simulink model "Z_Feedback"  (R2022b)
settings: Solver=FixedStepAuto  StartTime=0.0  StopTime=10.0  FixedStep=step_size  RelTol=1e-3
undefined symbols (not defined in the file): unicycle
libraries: simulink_extras x1
settings Model: Creator=Musta  LastModifiedBy=mustacchim

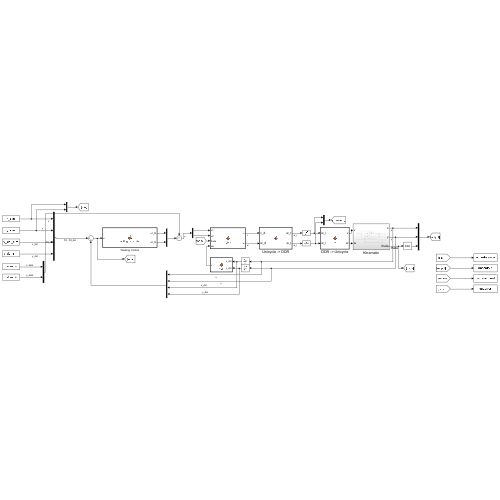
[thumbnail: Simulink's stored preview of the top-level diagram]
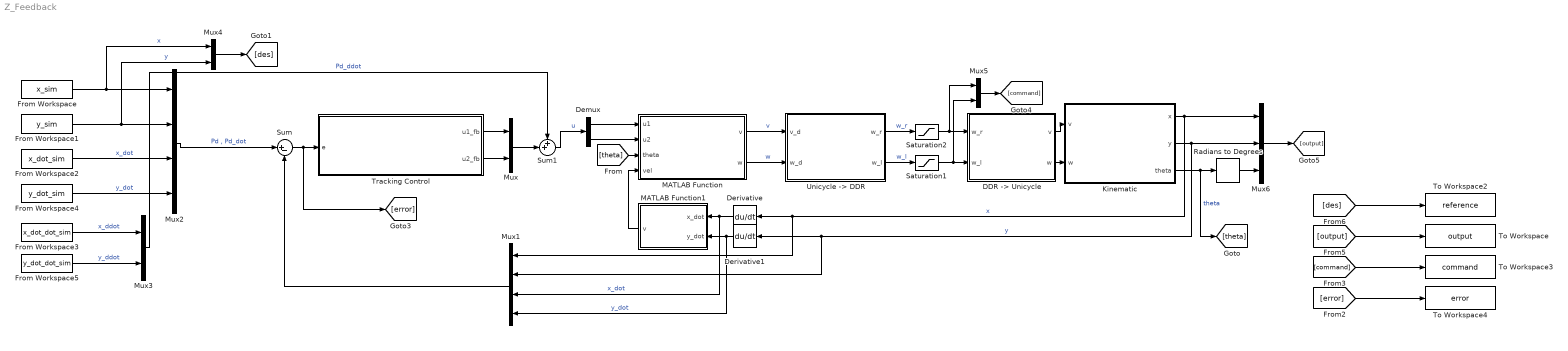
== system Z_Feedback ==
  " DDR -> Unicycle " : MATLAB Function  TreatAsAtomicUnit=on
  Demux : Demux  Outputs=2
  Derivative : Derivative
  Derivative1 : Derivative
  From Workspace : FromWorkspace  VariableName=x_sim
  From Workspace1 : FromWorkspace  VariableName=y_sim
  From Workspace2 : FromWorkspace  VariableName=x_dot_sim
  From Workspace3 : FromWorkspace  VariableName=x_dot_dot_sim
  From Workspace4 : FromWorkspace  VariableName=y_dot_sim
  From Workspace5 : FromWorkspace  VariableName=y_dot_dot_sim
  Kinematic : Subsystem
  MATLAB Function : MATLAB Function  TreatAsAtomicUnit=on
  MATLAB Function1 : MATLAB Function  TreatAsAtomicUnit=on
  Mux{,3..5} (4 alike) : Mux  Inputs=2
  Mux1 : Mux
  Mux2 : Mux
  Mux6 : Mux  Inputs=3
  Radians to Degrees : simulink_extras/Transformations/Radians to Degrees
  Saturation1 : Saturate  UpperLimit=unicycle.omegaWheelMax  LowerLimit=unicycle.omegaWheelMin
  Saturation2 : Saturate  UpperLimit=unicycle.omegaWheelMax  LowerLimit=unicycle.omegaWheelMin
  Sum : Sum  Inputs=|+-
  Sum1 : Sum  Inputs=++|
  To Workspace : ToWorkspace  VariableName=output  SaveFormat=Structure With Time  SampleTime=-1
  To Workspace2 : ToWorkspace  VariableName=reference  SaveFormat=Structure With Time  SampleTime=-1
  To Workspace3 : ToWorkspace  VariableName=command  SaveFormat=Structure With Time  SampleTime=-1
  To Workspace4 : ToWorkspace  VariableName=error  SaveFormat=Structure With Time  SampleTime=-1
  Tracking Control : MATLAB Function  TreatAsAtomicUnit=on
  "Unicycle -> DDR" : MATLAB Function  TreatAsAtomicUnit=on
  wires:
  Mux4/1 -> [des]
  Mux1/1 -> Sum/2
  Mux2/1 -> Sum/1  "Pd , Pd_dot"
  Demux/1 -> MATLAB Function/1(u1)
  Mux/1 -> Sum1/2
  Derivative1/1 -> Mux1/4, MATLAB Function1/2(y_dot)  "y_dot"
  From Workspace5/1 -> Mux3/2  "y_ddot"
  Derivative/1 -> Mux1/3, MATLAB Function1/1(x_dot)  "x_dot"
  Demux/2 -> MATLAB Function/2(u2)
  Tracking Control/2(u2_fb) -> Mux/2
  From Workspace1/1 -> Mux2/2, Mux4/2  "y"
  MATLAB Function1/1(v) -> MATLAB Function/4(vel)
  From Workspace3/1 -> Mux3/1  "x_ddot"
  Tracking Control/1(u1_fb) -> Mux/1
  MATLAB Function/1(v) -> "Unicycle -> DDR"/1(v_d)  "v"
  Sum1/1 -> Demux/1  "u"
  MATLAB Function/2(w) -> "Unicycle -> DDR"/2(w_d)  "w"
  From Workspace/1 -> Mux4/1, Mux2/1  "x"
  From Workspace2/1 -> Mux2/3  "x_dot"
  From Workspace4/1 -> Mux2/4  "y_dot"
  Mux3/1 -> Sum1/1  "Pd_ddot"
  Kinematic/3(theta) -> [theta], Radians to Degrees/1  "theta"
  Kinematic/1(x) -> Mux1/1, Derivative/1, Mux6/1  "x"
  " DDR -> Unicycle "/1(v) -> Kinematic/1(v)
  Radians to Degrees/1 -> Mux6/3
  Saturation2/1 -> " DDR -> Unicycle "/1(w_r), Mux5/1
  "Unicycle -> DDR"/1(w_r) -> Saturation2/1  "w_r"
  "Unicycle -> DDR"/2(w_l) -> Saturation1/1  "w_l"
  " DDR -> Unicycle "/2(w) -> Kinematic/2(w)
  Mux6/1 -> [output]
  Saturation1/1 -> Mux5/2, " DDR -> Unicycle "/2(w_l)
  Kinematic/2(y) -> Mux1/2, Derivative1/1, Mux6/2  "y"
  Mux5/1 -> [command]
  Sum/1 -> [error], Tracking Control/1(e)
  [theta] -> MATLAB Function/3(theta)
  [command] -> To Workspace3/1
  [output] -> To Workspace/1
  [des] -> To Workspace2/1
  [error] -> To Workspace4/1

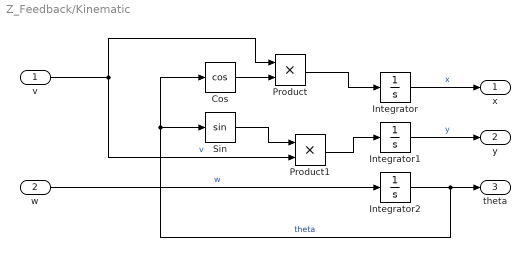
== system Z_Feedback/Kinematic ==
  v : Inport
  w : Inport  Port=2
  Cos : Trigonometry  Operator=cos
  Integrator : Integrator  InitialCondition=unicycle.ic.x
  Integrator1 : Integrator  InitialCondition=unicycle.ic.y
  Integrator2 : Integrator  InitialCondition=unicycle.ic.theta
  Product : Product
  Product1 : Product
  Sin : Trigonometry
  x : Outport
  y : Outport  Port=2
  theta : Outport  Port=3
  wires:
  w/1 -> Integrator2/1  "w"
  Product/1 -> Integrator/1
  v/1 -> Product/1, Product1/2  "v"
  Cos/1 -> Product/2
  Integrator1/1 -> y/1  "y"
  Integrator/1 -> x/1  "x"
  Integrator2/1 -> Cos/1, Sin/1, theta/1  "theta"
  Product1/1 -> Integrator1/1
  Sin/1 -> Product1/1

== matlab function Z_Feedback/MATLAB Function ==
  data: u1 input; u2 input; theta input; v output; w output; vel input
function [v,w] = T_inv(u1,u2,theta,vel)


if abs(vel) < 1e-3
    if abs(vel) >= 0
        vel = 1e-3;
    else 
        vel = -1e-3;
    end
end

T_i = [cos(theta) sin(theta);
      -sin(theta)/vel cos(theta)/vel];

v_w = T_i * [u1;u2];

v = v_w(1);
w = v_w(2);

== matlab function Z_Feedback/Tracking Control ==
  data: u1_fb output; u2_fb output; e input
function [u1_fb,u2_fb] = tracking_controller(e)

    %#codegen
    coder.extrinsic('evalin')
    k_p1 = 0;                  % Needed in order to set variable class correctly
    k_p2 = 0;                  % Needed in order to set variable class correctly
    k_d1 = 0;                  % Needed in order to set variable class correctly
    k_d2 = 0;                  % Needed in order to set variable class correctly
    k_p1 = evalin('base','k_p1'); % Read value from workspace
    k_p2 = evalin('base','k_p2'); % Read value from workspace
    k_d1 = evalin('base','k_d1'); % Read value from workspace
    k_d2 = evalin('base','k_d2'); % Read value from workspace

    e_x = e(1);
    e_y = e(2);
    e_xdot = e(3);
    e_ydot = e(4);
    
    % Controller
    u1_fb = k_p1 * e_x + k_d1 * e_xdot;
    u2_fb = k_p2 *e_y + k_d2 * e_ydot;

end

== matlab function Z_Feedback/MATLAB Function1 ==
  data: x_dot input; v output; y_dot input
function v = vel(x_dot,y_dot)

v = sqrt(x_dot^2 + y_dot^2);

== matlab function Z_Feedback/ DDR -> Unicycle  ==
  data: w_r input; v output; w_l input; w output
function [v, w] = fcn(w_r, w_l)

    %#codegen
    coder.extrinsic('evalin')
    d = 0;                  % Needed in order to set variable class correctly
    r = 0;                  % Needed in order to set variable class correctly
    d = evalin('base','unicycle.d'); % Read value from workspace
    r = evalin('base','unicycle.r'); % Read value from workspace

    v = r*(w_r + w_l)/2; % rad/s
    w = r*(w_r - w_l)/d; % rad/s

end

== matlab function Z_Feedback/Unicycle -> DDR ==
  data: v_d input; w_r output; w_d input; w_l output
function [w_r, w_l] = fcn(v_d, w_d)

    %#codegen
    coder.extrinsic('evalin')
    d = 0;                  % Needed in order to set variable class correctly
    r = 0;                  % Needed in order to set variable class correctly
    d = evalin('base','unicycle.d'); % Read value from workspace
    r = evalin('base','unicycle.r'); % Read value from workspace

    w_r = ((2 * v_d) + (w_d * d)) / (2 * r);
    w_l = ((2 * v_d) - (w_d * d)) / (2 * r);

end
